simulink model "generator_noload_ssc"  (R2014a)
settings: Solver=ode23t  StartTime=0.0  StopTime=8  MaxStep=1e-4  RelTol=1e-4
undefined symbols (not defined in the file or in its folder): j, pe
libraries: fl_lib x26, pe_lib x9, nesl_utility x7, simulink_extras x2
CloseFcn:
  | if exist( 'h1_pe_sm_control', 'var' ) && ishandle( h1_pe_sm_control )
  |     delete( h1_pe_sm_control );
  | end
Description:
  | Three-Phase Synchronous Machine Control
  | 
  | This example shows how to control and initialize a Synchronous Machine (SM).
  | 
  | The test circuit shows the SM being used as a generator, the terminal voltage is controlled using an AVR, and the speed is controlled using a governor.
  | To view the SM machine base values and initial conditions, right-click on the SM block and select 'Power Systems', 'Synchronous Machine',  and then 'Display Base Values', 'Display Associated Base Values', or 'Associated Initial Conditions'.
  | The overall model has been initialized to start in periodic steady state to supply a load of  250MW/15MVAr.
  | 
  | 
  | Copyright 2008-2014 The MathWorks, Inc.
settings Model: Creator=MathWorks  LastModifiedBy=cosorio
settings DataIOCC: LimitDataPoints=off  SaveOutput=off  SignalLogging=off  DSMLogging=off  SaveTime=off
settings DebuggingCC: UnderspecifiedInitializationDetection=Classic
settings SimscapeCC: SimscapeLogType=all  SimscapeLogSimulationStatistics=on  SimscapeLogName=smnoload_simlog  SimscapeLogLimitData=off

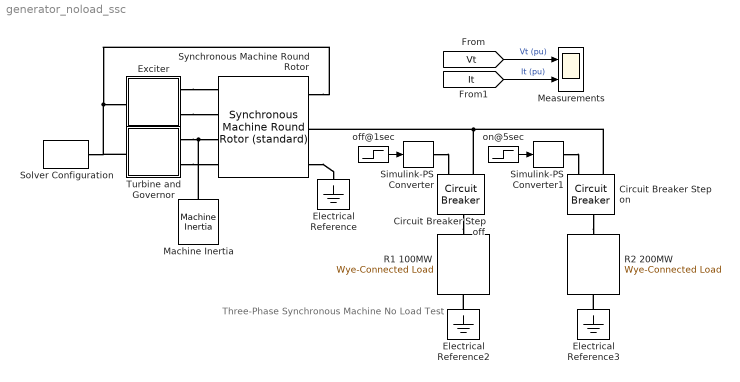
== system generator_noload_ssc ==
  note: Three-Phase Synchronous Machine
      | No Load Test
  Circuit Breaker Step off : pe_lib/Switches & Breakers/Circuit Breaker  R_closed=0.001 Ohm  G_open=1e-4 1/Ohm  threshold=0.5 V  initial_state=1
  Circuit Breaker Step on : pe_lib/Switches & Breakers/Circuit Breaker  R_closed=0.001 Ohm  G_open=1e-4 1/Ohm  threshold=0.5 V  initial_state=0
  Electrical Reference : fl_lib/Electrical/Electrical Elements/Electrical Reference
  Electrical Reference2 : fl_lib/Electrical/Electrical Elements/Electrical Reference
  Electrical Reference3 : fl_lib/Electrical/Electrical Elements/Electrical Reference
  Exciter : Subsystem
  Machine Inertia : pe_lib/Machines/Machine Inertia  SRated=555e6 V*A  FRated=60 Hz  nPolePairs=1  inertia_option=2  J=27548 kg*m^2  H=3.525 s*W/V/A  damper_option=2  D=39.0509 N*m/(rad/s)  pu_D=0.01  initialization_option=2  fMechanical0=60 Hz  fElectrical0=60 Hz
  Measurements : Scope  NumInputPorts=2
      settings: YMin=0.2~0  YMax=1.2~0.5
  R1 100MW : pe_lib/Passive Devices/Wye-Connected Load  parameterization=2  component_structure=1  component_structure_PQ=1  R=1 Ohm  L=0.001 H  C=1e-6 F  IL0=[ 0 0 0 ] A  VC0=[ 0 0 0 ] V  R_parasitic=1e-6 Ohm  G_parasitic=1e-6 1/Ohm  VRated=24e3 V  FRated=60 Hz  P=100e6 W  Qpos=10e6 V*A  Qneg=-100 V*A  Vmag0=2.4e+4 V  Vang0=0 deg  Freq0=60 Hz  R_parasitic_PQ=1e-6 Ohm  G_parasitic_PQ=1e-6 1/Ohm
  R2 200MW : pe_lib/Passive Devices/Wye-Connected Load  parameterization=2  component_structure=1  component_structure_PQ=1  R=1 Ohm  L=0.001 H  C=1e-6 F  IL0=[ 0 0 0 ] A  VC0=[ 0 0 0 ] V  R_parasitic=1e-6 Ohm  G_parasitic=1e-6 1/Ohm  VRated=24e3 V  FRated=60 Hz  P=200e6 W  Qpos=20e6 V*A  Qneg=-100 V*A  Vmag0=0 V  Vang0=0 deg  Freq0=60 Hz  R_parasitic_PQ=1e-6 Ohm  G_parasitic_PQ=1e-6 1/Ohm
  Simulink-PS Converter : nesl_utility/Simulink-PS Converter  PhysicalDomain=network_engine_domain  SubClassName=ps_input  LeftPortType=input  RightPortType=output  PseudoPeriodic=off  Frequencies=[]  NoiseDistribution=none  NoiseParameters=[]  Unit=1  AffineConversion=off  InputFiltering=off  SimscapeFilterOrder=1  InputFilterTimeConstant=0.001  UdotUserProvided=1
  Simulink-PS Converter1 : nesl_utility/Simulink-PS Converter  PhysicalDomain=network_engine_domain  SubClassName=ps_input  LeftPortType=input  RightPortType=output  PseudoPeriodic=off  Frequencies=[]  NoiseDistribution=none  NoiseParameters=[]  Unit=1  AffineConversion=off  InputFiltering=off  SimscapeFilterOrder=1  InputFilterTimeConstant=0.001  UdotUserProvided=1
  Solver Configuration : nesl_utility/Solver Configuration  PhysicalDomain=network_engine_domain  SubClassName=solver  LeftPortType=input  RightPortType=generic  Accelerate=off  Tones=[]  Harmonics=[]  SimulateNoise=off  Profile=off  UseLocalSampling=off  EnableSwitchedLinearOptims=on  FrequencyDomain=off  UseCCode=off  RelTol=0.001  AbsTol=1e-06  MinStep=1e-09  ToWorkspace=off  DoDC=off  ResidualTolerance=1e-09  UseLocalSolver=on  LocalSolverChoice=NE_BACKWARD_EULER_ADVANCER  LocalSolverSampleTime=1e-4  DoFixedCost=on  MaxNonlinIter=5  MaxModeIter=2  LinearAlgebra=Sparse  DelaysMemoryBudget=1024  AutomaticFiltering=off  FilteringTimeConstant=0.001
  Synchronous Machine Round Rotor : pe_lib/Machines/Synchronous Machine (Round Rotor)/Synchronous Machine Round Rotor (standard)  SRated=555e6 V*A  VRated=24e3 V  FRated=60 Hz  nPolePairs=1  fieldCircuitParameterization_option=2  baseEfd=92.95 V  baseIfd=1300 A  Ra=0.003  Xl=0.15  Xd=1.81  Xq=1.76  X0=0  Xdd=0.3  Xqd=0.65  Xddd=0.23  Xqdd=0.25  d_transient_option=1  Td0d=8 s  Tdd=1.3260 s  d_subtransient_option=1  Td0dd=0.03 s  Tddd=0.0230 s  q_transient_option=1  Tq0d=1 s  Tqd=0.3693 s  q_subtransient_option=1  Tq0dd=0.07 s  Tqdd=0.0269 s  saturation_option=0  saturation_ifd=[0.00, 0.48, 0.76, 1.38, 1.79]  saturation_Vag=[0.00, 0.80, 1.08, 1.31, 1.40]  initialization_option=2  angular_position0=0 deg  pu_psid0=0  pu_psiq0=0  pu_psi00=0  pu_psifd0=0  pu_psi1d0=0  pu_psi1q0=0  pu_psi2q0=0  Vmag0=24e3 V  Vang0=17.5858 deg  Pt0=100e6 V*A  Qt0=0 V*A  shift_3ph=[nan, nan, nan] rad  connection_option=int32(pe.Connection.wye)  num_q_dampers=2  oneOverOmega=nan s/rad  L0=nan  Ladu=nan  Laqu=nan  Ll=nan  Lfd=nan  Rfd=nan  L1d=nan  R1d=nan  L1q=nan  R1q=nan  L2q=nan  R2q=nan  Xmin=1e-9  base_v=nan V  base_i=nan A  base_torque=nan N*m  base_wMechanical=nan rad/s  base_rc_efd=nan V  base_rc_ifd=nan A  base_fd_Efd=nan V  base_fd_Ifd=nan A  saturation_psi=0  saturation_K_s=1
  "Turbine and Governor " : Subsystem  mask(Governor and Prime Mover){pu_speed_reference=1, droop_percentage=5, pu_load_reference_setpoint=0.8, T_G=0.01, T_CH=0.05, base_torque=265402, pu_torque0=0.180278}
      mask prompts: pu_speed_reference "Speed reference, (pu)"; droop_percentage "Percentage droop, (%)"; pu_load_reference_setpoint "Load reference setpoint, (pu)"; T_G "Time constant of governor, (s)"; T_CH "Time constant of main inlet volumes and steam chest, (s)"; base_torque "Base torque, (N*m)"; pu_torque0 "Initial torque, (pu)"
      mask help:
      | Implements a synchronous machine governor and prime mover. The prime mover is a non-reheat steam turbine.
      |
      | The input to the block is a per-unit synchronous machine measurement vector.
      |
      | R and C are mechanical rotational ports.
  off@1sec : Step  SampleTime=0
  on@5sec : Step  Time=5  Before=1  After=0  SampleTime=0
  wires:
  off@1sec/1 -> Simulink-PS Converter/1
  on@5sec/1 -> Simulink-PS Converter1/1
  [Vt] -> Measurements/1  "Vt (pu)"
  [It] -> Measurements/2  "It (pu)"
  connections:
  Circuit Breaker Step on/LConn2 -- Circuit Breaker Step off/LConn2 -- Synchronous Machine Round Rotor/RConn2
  Exciter/RConn1 -- Synchronous Machine Round Rotor/LConn1
  Synchronous Machine Round Rotor/RConn1 -- "Turbine and Governor "/LConn1 -- Solver Configuration/RConn1 -- Exciter/LConn1
  Exciter/RConn2 -- Synchronous Machine Round Rotor/LConn2
  Synchronous Machine Round Rotor/RConn3 -- Electrical Reference/LConn1
  "Turbine and Governor "/RConn2 -- Synchronous Machine Round Rotor/LConn4
  "Turbine and Governor "/RConn1 -- Synchronous Machine Round Rotor/LConn3 -- Machine Inertia/LConn1
  Electrical Reference2/LConn1 -- R1 100MW/RConn1
  Circuit Breaker Step off/RConn1 -- R1 100MW/LConn1
  Simulink-PS Converter/RConn1 -- Circuit Breaker Step off/LConn1
  Simulink-PS Converter1/RConn1 -- Circuit Breaker Step on/LConn1
  Circuit Breaker Step on/RConn1 -- R2 200MW/LConn1
  Electrical Reference3/LConn1 -- R2 200MW/RConn1

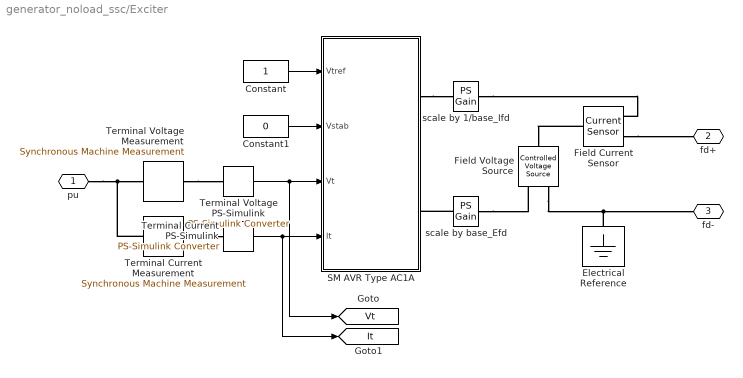
== system generator_noload_ssc/Exciter ==
  Constant : Constant
  Constant1 : Constant  Value=0
  Electrical Reference : fl_lib/Electrical/Electrical Elements/Electrical Reference
  Field Current Sensor : fl_lib/Electrical/Electrical Sensors/Current Sensor
  Field Voltage Source : fl_lib/Electrical/Electrical Sources/Controlled Voltage Source
  SM AVR Type AC1A : Subsystem  mask(AVR and Excitation System){RcXc=[0 0], Tr=20e-3, KaTa=[400 0.02], KeTe=[1 0.8], TbTc=[0 0], KfTf=[0.03 1], Ve21=[3.14 4.18], SeVe21=[0.03 0.1], Vaminmax=[-14.5 14.5], Vrminmax=[-5.43 6.03], Kc=0.2, Kd=0.38, v0=[1,1.05231]}
      mask prompts: RcXc "Compensation resistance and reactance, [Rc(pu)  Xc(pu)]:"; Tr "Voltage sensing and compensation time constant, Tr(s):"; KaTa "Voltage regulator gain and time constant, [Ka Ta(s)]:"; KeTe "Exciter field gain and time constant, [Ke Te(s)]:"; TbTc "Transient gain reduction lag and lead time constants, [Tb(s) Tc(s)]:"; KfTf "Damping filter gain and time constant, [Kf  Tf(s)]:"; Ve21 "Field voltage values, [Ve2(pu) Ve1(pu)]:"; SeVe21 "Saturation values, [SeVe2(pu) SeVe1(pu)]:"; Vaminmax "Regulator internal voltage limits, [Vamin(pu) Vamax(pu)]:"; Vrminmax "Voltage regulator output limits, [Vrmin(pu) Vrmax(pu)]:"; Kc "Rectifier regulation factor, Kc(pu):"; Kd "Exciter internal reactance, Kd(pu):"; v0 "Initial terminal voltage and initial field voltage, [Vt0(pu) Efd0(pu)]:"
      mask help:
      | Implements an AC1A synchronous machine Automatic Voltage Regulator (AVR) combined with an exciter.
      |
      | The inputs to the block are per-unit voltages and current.
      |
      | The output of the block is the per-unit field voltage (Efd(pu)).
      mask init:
      | Rc=RcXc(1);Xc=RcXc(2);
      | Ka=KaTa(1);Ta=KaTa(2);
      | Ke=KeTe(1);Te=KeTe(2);
      | Tb=TbTc(1);Tc=TbTc(2);
      | Vamin=Vaminmax(1);Vamax=Vaminmax(2);
      | Vrmin=Vrminmax(1);Vrmax=Vrminmax(2);
      | Kf=KfTf(1);Tf=KfTf(2);
      | Ve2=Ve21(1);Ve1=Ve21(2);
      | SeVe2=SeVe21(1);SeVe1=SeVe21(2);
      | Vt0=v0(1);Efd0=v0(2);
      | 
      | % initialisation
      | x0_exc=Efd0*(1+Kc*0.577);
      | 
      | Vfe0 = interp1( [0 Ve2 Ve1], [0 SeVe2 SeVe1], x0_exc )...
      |     + Ke*x0_exc...
      |     + Kd*Efd0;
      | 
      | gap = 1e-1;
      | Fex_xData = 0:gap:1+gap;
      | 
      | mode1Idx = Fex_xData <= 0.433;
      | mode2Idx = (0.433 < Fex_xData) & (Fex_xData < 0.75);
      | mode3Idx = (0.75 <= Fex_xData) & (Fex_xData <= 1);
      | mode4Idx = 1 < Fex_xData;
      | 
      | Fex_yData = zeros( size( Fex_xData ) );
      | Fex_yData( mode1Idx ) = 1 - 0.577.*Fex_xData( mode1Idx );
      | Fex_yData( mode2Idx ) = sqrt( 0.75 - Fex_xData( mode2Idx ).^2 );
      | Fex_yData( mode3Idx ) = 1.732*( 1 - Fex_xData( mode3Idx ) );
      | Fex_yData( mode4Idx ) = 0;
      | 
      | clear( 'gap', 'mode1Idx', 'mode2Idx',  'mode3Idx',  'mode4Idx' );
  Terminal Current Measurement : pe_lib/Machines/Synchronous Machine Measurement  output_idx=15
  Terminal Current PS-Simulink : nesl_utility/PS-Simulink Converter  PhysicalDomain=network_engine_domain  SubClassName=ps_output  LeftPortType=input  RightPortType=output  PseudoPeriodic=off  Frequencies=[]  Unit=1  AffineConversion=off
  Terminal Voltage Measurement : pe_lib/Machines/Synchronous Machine Measurement  output_idx=14
  Terminal Voltage PS-Simulink : nesl_utility/PS-Simulink Converter  PhysicalDomain=network_engine_domain  SubClassName=ps_output  LeftPortType=input  RightPortType=output  PseudoPeriodic=off  Frequencies=[]  Unit=1  AffineConversion=off
  scale by 1/base_Ifd : fl_lib/Physical Signals/Functions/PS Gain  gain=1/1368.01
  scale by base_Efd : fl_lib/Physical Signals/Functions/PS Gain  gain=98.65
  pu : PMIOPort  Port=1  Side=Left
  fd+ : PMIOPort  Port=2  Side=Right
  fd- : PMIOPort  Port=3  Side=Right
  tag scope: It=global, Vt=global
  wires:
  Constant/1 -> SM AVR Type AC1A/1(Vtref)
  Constant1/1 -> SM AVR Type AC1A/2(Vstab)
  Terminal Voltage PS-Simulink/1 -> [Vt], SM AVR Type AC1A/3(Vt)
  Terminal Current PS-Simulink/1 -> [It], SM AVR Type AC1A/4(It)
  connections:
  Field Voltage Source/RConn2 -- Electrical Reference/LConn1 -- fd-/RConn1
  Field Current Sensor/RConn2 -- fd+/RConn1
  Field Current Sensor/LConn1 -- Field Voltage Source/LConn1
  scale by 1/base_Ifd/LConn1 -- Field Current Sensor/RConn1
  scale by base_Efd/RConn1 -- Field Voltage Source/RConn1
  scale by base_Efd/LConn1 -- SM AVR Type AC1A/RConn2
  SM AVR Type AC1A/RConn1 -- scale by 1/base_Ifd/RConn1
  Terminal Current Measurement/RConn1 -- Terminal Current PS-Simulink/LConn1
  Terminal Voltage Measurement/RConn1 -- Terminal Voltage PS-Simulink/LConn1
  pu/RConn1 -- Terminal Current Measurement/LConn1 -- Terminal Voltage Measurement/LConn1

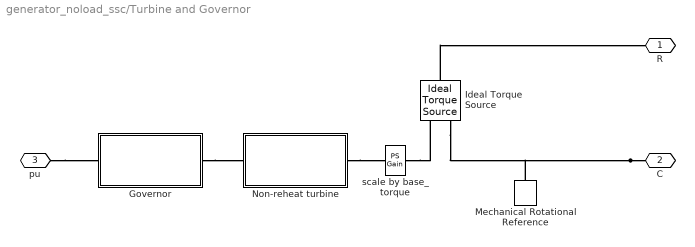
== system generator_noload_ssc/Turbine and Governor  ==
  Governor : Subsystem
  Ideal Torque Source : fl_lib/Mechanical/Mechanical Sources/Ideal Torque Source
  Mechanical Rotational Reference : fl_lib/Mechanical/Rotational Elements/Mechanical Rotational Reference
  Non-reheat turbine : Subsystem
  scale by base_torque : fl_lib/Physical Signals/Functions/PS Gain  gain=base_torque
  R : PMIOPort  Port=1  Side=Right
  C : PMIOPort  Port=2  Side=Right
  pu : PMIOPort  Port=3  Side=Left
  connections:
  C/RConn1 -- Ideal Torque Source/RConn2 -- Mechanical Rotational Reference/LConn1
  Ideal Torque Source/LConn1 -- R/RConn1
  Governor/RConn1 -- Non-reheat turbine/LConn1
  pu/RConn1 -- Governor/LConn1
  scale by base_torque/RConn1 -- Ideal Torque Source/RConn1
  Non-reheat turbine/RConn1 -- scale by base_torque/LConn1

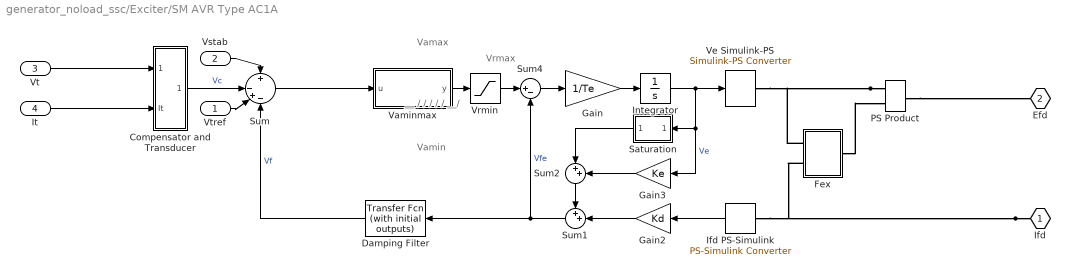
== system generator_noload_ssc/Exciter/SM AVR Type AC1A ==
  note: Vrmax
  note: Vamax
  note: Vamin
  note: __
      |               /
      |             /
      |           /
      |         /
      |       /
      | __/
  Vtref : Inport
  Vstab : Inport  Port=2
  Vt : Inport  Port=3
  It : Inport  Port=4
  Compensator and Transducer : Subsystem  mask{RcXc=[Rc Xc], Tr=Tr}
      mask prompts: RcXc "Compensation resistance and reactance, [Rc(pu)  Xc(pu)]:"; Tr "Voltage sensing and compensation time constant, Tr(s):"
      mask init:
      | Rc=RcXc(1);Xc=RcXc(2);
  Damping Filter : simulink_extras/Additional Linear/Transfer Fcn (with initial outputs)  N=[Kf 0]  D=[Tf 1]  Y0=-Vfe0/Ka  U0=Vfe0
  Fex : Subsystem  mask{Kc=Kc}
      mask prompts: Kc "Rectifier regulation factor, Kc(pu):"
  Gain : Gain  Gain=1/Te  SaturateOnIntegerOverflow=on  OutDataTypeStr=Inherit: Same as input  ParamDataTypeStr=Inherit: Same as input
  Gain2 : Gain  Gain=Kd  SaturateOnIntegerOverflow=on  OutDataTypeStr=Inherit: Same as input  ParamDataTypeStr=Inherit: Same as input
  Gain3 : Gain  Gain=Ke  SaturateOnIntegerOverflow=on  OutDataTypeStr=Inherit: Same as input  ParamDataTypeStr=Inherit: Same as input
  Ifd PS-Simulink : nesl_utility/PS-Simulink Converter  PhysicalDomain=network_engine_domain  SubClassName=ps_output  LeftPortType=input  RightPortType=output  PseudoPeriodic=off  Frequencies=[]  Unit=1  AffineConversion=off
  Integrator : Integrator  InitialCondition=x0_exc  LimitOutput=on  LowerSaturationLimit=0
  PS Product : fl_lib/Physical Signals/Functions/PS Product
  Saturation : Subsystem  mask{Ve21=[Ve2 Ve1], SeVe21=[SeVe2 SeVe1]}
      mask prompts: Ve21 "Field voltage values, [Ve2(pu) Ve1(pu)]:"; SeVe21 "Saturation values, [SeVe2(pu) SeVe1(pu)]:"
      mask init:
      | Ve2=Ve21(1);Ve1=Ve21(2);
      | SeVe2=SeVe21(1);SeVe1=SeVe21(2);
  Sum : Sum  Inputs=+|-+-  SaturateOnIntegerOverflow=on  InputSameDT=on  OutDataTypeStr=Inherit: Same as first input
  Sum1 : Sum  Inputs=++|  SaturateOnIntegerOverflow=on  InputSameDT=on  OutDataTypeStr=Inherit: Same as first input
  Sum2 : Sum  Inputs=|++  SaturateOnIntegerOverflow=on  InputSameDT=on  OutDataTypeStr=Inherit: Same as first input
  Sum4 : Sum  Inputs=|+-  SaturateOnIntegerOverflow=on  InputSameDT=on  OutDataTypeStr=Inherit: Same as first input
  Vaminmax : Subsystem  mask{Ka=Ka, Ta=Ta, Vaminmax=[Vamin Vamax], X0=Vfe0}
      mask prompts: Ka "Voltage regulator gain, Ka"; Ta "Voltage regulator time constant, Ta(s)"; Vaminmax "Regulator internal voltage limits, [Vamin(pu) Vamax(pu)]:"; X0 "Initial conditions:"
      mask init:
      | Vamin=Vaminmax(1);Vamax=Vaminmax(2);
      mask Display: dpoly([Ka],[Ta 1],'s')
  "Ve Simulink-PS " : nesl_utility/Simulink-PS Converter  PhysicalDomain=network_engine_domain  SubClassName=ps_input  LeftPortType=input  RightPortType=output  PseudoPeriodic=off  Frequencies=[]  NoiseDistribution=none  NoiseParameters=[]  Unit=1  AffineConversion=off  InputFiltering=off  SimscapeFilterOrder=1  InputFilterTimeConstant=.001  UdotUserProvided=[]
  Vrmin : Saturate  UpperLimit=Vrmax  LowerLimit=Vrmin
  Ifd : PMIOPort  Port=1  Side=Right
  Efd : PMIOPort  Port=2  Side=Right
  wires:
  Ifd PS-Simulink/1 -> Gain2/1
  Vt/1 -> Compensator and Transducer/1(Vt)
  Vtref/1 -> Sum/3
  Vstab/1 -> Sum/1
  Damping Filter/1 -> Sum/4  "Vf"
  Vrmin/1 -> Sum4/1
  Sum1/1 -> Sum4/2, Damping Filter/1  "Vfe"
  Gain/1 -> Integrator/1
  Integrator/1 -> Saturation/1(Ve), Gain3/1, "Ve Simulink-PS "/1  "Ve"
  Sum2/1 -> Sum1/1
  Gain2/1 -> Sum1/2
  Gain3/1 -> Sum2/2
  Saturation/1(Vx) -> Sum2/1
  It/1 -> Compensator and Transducer/2(It)
  Sum4/1 -> Gain/1
  Vaminmax/1(y) -> Vrmin/1
  Sum/1 -> Vaminmax/1(u)
  Compensator and Transducer/1(Vc) -> Sum/2  "Vc"
  connections:
  Ifd/RConn1 -- Fex/LConn2 -- Ifd PS-Simulink/LConn1
  PS Product/RConn1 -- Efd/RConn1
  PS Product/LConn1 -- Fex/LConn1 -- "Ve Simulink-PS "/RConn1
  Fex/RConn1 -- PS Product/LConn2

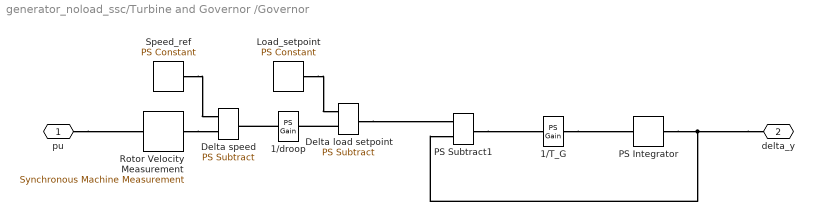
== system generator_noload_ssc/Turbine and Governor /Governor ==
  1/T_G : fl_lib/Physical Signals/Functions/PS Gain  gain=1/T_G
  1/droop : fl_lib/Physical Signals/Functions/PS Gain  gain=1/(droop_percentage/100)
  Delta load setpoint : fl_lib/Physical Signals/Functions/PS Subtract
  Delta speed : fl_lib/Physical Signals/Functions/PS Subtract
  Load_setpoint : fl_lib/Physical Signals/Sources/PS Constant  constant=pu_load_reference_setpoint
  PS Integrator : fl_lib/Physical Signals/Linear Operators/PS Integrator  x0=pu_torque0
  PS Subtract1 : fl_lib/Physical Signals/Functions/PS Subtract
  Rotor Velocity Measurement : pe_lib/Machines/Synchronous Machine Measurement  output_idx=4
  Speed_ref : fl_lib/Physical Signals/Sources/PS Constant  constant=pu_speed_reference
  pu : PMIOPort  Port=1  Side=Left
  delta_y : PMIOPort  Port=2  Side=Right
  connections:
  delta_y/RConn1 -- PS Subtract1/LConn2 -- PS Integrator/RConn1
  PS Subtract1/RConn1 -- 1/T_G/LConn1
  1/T_G/RConn1 -- PS Integrator/LConn1
  Load_setpoint/RConn1 -- Delta load setpoint/LConn1
  1/droop/LConn1 -- Delta speed/RConn1
  Speed_ref/RConn1 -- Delta speed/LConn2
  Rotor Velocity Measurement/RConn1 -- Delta speed/LConn1
  Delta load setpoint/LConn2 -- 1/droop/RConn1
  Delta load setpoint/RConn1 -- PS Subtract1/LConn1
  pu/RConn1 -- Rotor Velocity Measurement/LConn1

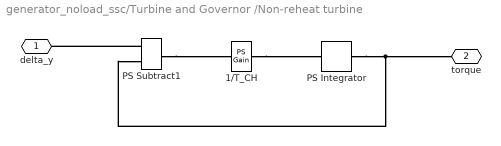
== system generator_noload_ssc/Turbine and Governor /Non-reheat turbine ==
  1/T_CH : fl_lib/Physical Signals/Functions/PS Gain  gain=1/T_CH
  PS Integrator : fl_lib/Physical Signals/Linear Operators/PS Integrator  x0=pu_torque0
  PS Subtract1 : fl_lib/Physical Signals/Functions/PS Subtract
  delta_y : PMIOPort  Port=1  Side=Left
  torque : PMIOPort  Port=2  Side=Right
  connections:
  1/T_CH/RConn1 -- PS Integrator/LConn1
  PS Subtract1/LConn1 -- delta_y/RConn1
  PS Subtract1/RConn1 -- 1/T_CH/LConn1
  PS Integrator/RConn1 -- PS Subtract1/LConn2 -- torque/RConn1

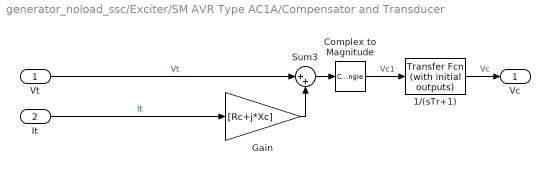
== system generator_noload_ssc/Exciter/SM AVR Type AC1A/Compensator and Transducer ==
  Vt : Inport
  It : Inport  Port=2
  1/(sTr+1) : simulink_extras/Additional Linear/Transfer Fcn (with initial outputs)  N=1  D=[Tr 1]  Y0=Vt0  U0=Vt0
  Complex to Magnitude : ComplexToMagnitudeAngle  Output=Magnitude
  Gain : Gain  Gain=[Rc+j*Xc]  SaturateOnIntegerOverflow=on  OutDataTypeStr=Inherit: Same as input  ParamDataTypeStr=Inherit: Same as input
  Sum3 : Sum  Inputs=|++  SaturateOnIntegerOverflow=on  InputSameDT=on  OutDataTypeStr=Inherit: Same as first input
  Vc : Outport
  wires:
  Vt/1 -> Sum3/1  "Vt"
  It/1 -> Gain/1  "It"
  Gain/1 -> Sum3/2
  Sum3/1 -> Complex to Magnitude/1
  Complex to Magnitude/1 -> 1/(sTr+1)/1  "Vc1"
  1/(sTr+1)/1 -> Vc/1  "Vc"

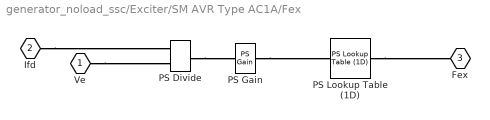
== system generator_noload_ssc/Exciter/SM AVR Type AC1A/Fex ==
  PS Divide : fl_lib/Physical Signals/Functions/PS Divide
  PS Gain : fl_lib/Physical Signals/Functions/PS Gain  gain=Kc
  PS Lookup Table (1D) : fl_lib/Physical Signals/Lookup Tables/PS Lookup Table (1D)  x_t=Fex_xData  y_t=Fex_yData  interp_method=1  extrap_method=1
  Ve : PMIOPort  Port=1  Side=Left
  Ifd : PMIOPort  Port=2  Side=Left
  Fex : PMIOPort  Port=3  Side=Right
  connections:
  PS Lookup Table (1D)/RConn1 -- Fex/RConn1
  PS Gain/RConn1 -- PS Lookup Table (1D)/LConn1
  PS Divide/RConn1 -- PS Gain/LConn1
  Ve/RConn1 -- PS Divide/LConn2
  Ifd/RConn1 -- PS Divide/LConn1

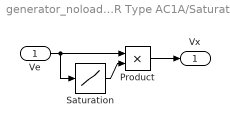
== system generator_noload_ssc/Exciter/SM AVR Type AC1A/Saturation ==
  Ve : Inport
  Product : Product  SaturateOnIntegerOverflow=on  RndMeth=Zero  InputSameDT=on  OutDataTypeStr=Inherit: Same as first input
  Saturation : Lookup  InputValues=[0 Ve2 Ve1]  Table=[0 SeVe2 SeVe1]  SaturateOnIntegerOverflow=on
  Vx : Outport
  wires:
  Ve/1 -> Product/1, Saturation/1
  Saturation/1 -> Product/2
  Product/1 -> Vx/1

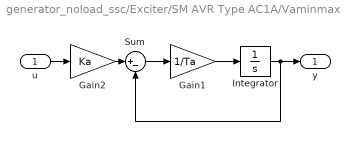
== system generator_noload_ssc/Exciter/SM AVR Type AC1A/Vaminmax ==
  u : Inport
  Gain1 : Gain  Gain=1/Ta  SaturateOnIntegerOverflow=on  OutDataTypeStr=Inherit: Same as input  ParamDataTypeStr=Inherit: Same as input
  Gain2 : Gain  Gain=Ka  SaturateOnIntegerOverflow=on  OutDataTypeStr=Inherit: Same as input  ParamDataTypeStr=Inherit: Same as input
  Integrator : Integrator  InitialCondition=X0  LimitOutput=on  UpperSaturationLimit=Vamax  LowerSaturationLimit=Vamin
  Sum : Sum  Inputs=|+-  SaturateOnIntegerOverflow=on  InputSameDT=on  OutDataTypeStr=Inherit: Same as first input
  y : Outport
  wires:
  u/1 -> Gain2/1
  Sum/1 -> Gain1/1
  Integrator/1 -> y/1, Sum/2
  Gain2/1 -> Sum/1
  Gain1/1 -> Integrator/1
